simulink model "InjSys_CtlQnt1"  (R2016b)
settings: configuration reference "CodeGenConfigSet" (kept outside this file)
libraries: simulink x2
settings Model: Creator=lenovo  LastModifiedBy=mayongchao
settings ConfigSetRef: SourceLocation=Base Workspace

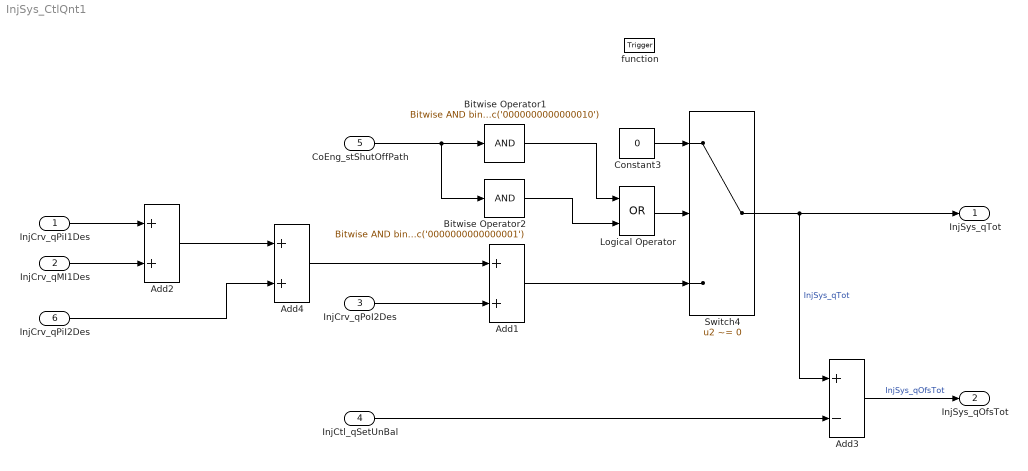
== system InjSys_CtlQnt1 ==
  InjCrv_qPiI1Des : Inport  Tag=mg/hub  Description=Desired PiI injection quantity  OutMin=-319  OutMax=319  OutDataTypeStr=FuelMass_mg_hub
  InjCrv_qMI1Des : Inport  Tag=mg/hub  Description=desired MI1 injection quantity  Port=2  OutMin=-319  OutMax=319  OutDataTypeStr=FuelMass_mg_hub
  InjCrv_qPoI2Des : Inport  Tag=mg/hub  Description=Desired PoI2 injection quantity  Port=3  OutMin=-319  OutMax=319  OutDataTypeStr=FuelMass_mg_hub
  InjCtl_qSetUnBal : Inport  Tag=mg/hub  Description=Current injection quantity  Port=4  OutMin=-319  OutMax=319  OutDataTypeStr=FuelMass_mg_hub
  CoEng_stShutOffPath : Inport  Description=Active shut-off paths resulting from active reversible,irreversible and afterrun shut-off paths  Port=5  OutMin=0  OutMax=65535  OutDataTypeStr=State_uint16
  InjCrv_qPiI2Des : Inport  Tag=mg/hub  Description=Desired PiI injection quantity  Port=6  OutMin=-319  OutMax=319  OutDataTypeStr=FuelMass_mg_hub
  function : TriggerPort  TriggerType=function-call  VariantControl=Variant
  Add1 : Sum  OutDataTypeStr=Inherit: Inherit via back propagation  SaturateOnIntegerOverflow=on  InputSameDT=on
  Add2 : Sum  OutDataTypeStr=Inherit: Inherit via back propagation  SaturateOnIntegerOverflow=on  InputSameDT=on
  Add3 : Sum  Inputs=+-  OutDataTypeStr=Inherit: Inherit via back propagation  SaturateOnIntegerOverflow=on  InputSameDT=on
  Add4 : Sum  OutDataTypeStr=Inherit: Inherit via back propagation  SaturateOnIntegerOverflow=on  InputSameDT=on
  Bitwise Operator1 : simulink/Logic and Bit Operations/Bitwise Operator  logicop=AND  UseBitMask=on  BitMask=bin2dec('0000000000000010')  BitMaskRealWorld=Stored Integer
  Bitwise Operator2 : simulink/Logic and Bit Operations/Bitwise Operator  logicop=AND  UseBitMask=on  BitMask=bin2dec('0000000000000001')  BitMaskRealWorld=Stored Integer
  Constant3 : Constant  Value=0  OutDataTypeStr=Inherit: Inherit via back propagation
  Logical Operator : Logic  Operator=OR  AllPortsSameDT=off  OutDataTypeStr=boolean
  Switch4 : Switch  Criteria=u2 ~= 0  SaturateOnIntegerOverflow=on  InputSameDT=on
  InjSys_qTot : Outport  Tag=mg/hub  Description=Total engine injection quantity  OutMin=-319  OutMax=319  OutDataTypeStr=FuelMass_mg_hub
  InjSys_qOfsTot : Outport  Tag=mg/hub  Description=Non-torque generating quantity, the offset-quantity from torque generating quantity to total quantity  Port=2  OutMin=-319  OutMax=319  OutDataTypeStr=FuelMass_mg_hub
  wires:
  InjCrv_qMI1Des/1 -> Add2/2
  InjCrv_qPoI2Des/1 -> Add1/2
  InjCrv_qPiI1Des/1 -> Add2/1
  Bitwise Operator1/1 -> Logical Operator/1
  Bitwise Operator2/1 -> Logical Operator/2
  Logical Operator/1 -> Switch4/2
  CoEng_stShutOffPath/1 -> Bitwise Operator1/1, Bitwise Operator2/1
  Constant3/1 -> Switch4/1
  Add2/1 -> Add4/1
  Add1/1 -> Switch4/3
  Add3/1 -> InjSys_qOfsTot/1  "InjSys_qOfsTot"
  Switch4/1 -> InjSys_qTot/1, Add3/1  "InjSys_qTot"
  InjCtl_qSetUnBal/1 -> Add3/2
  Add4/1 -> Add1/1
  InjCrv_qPiI2Des/1 -> Add4/2
